simulink model "four_2"  (R2018a)
settings: Solver=VariableStepAuto  StartTime=0.0  StopTime=0.1  RelTol=1e-3
libraries: powerlib x17, powerlib_extras x1
settings Model: Creator=14064  LastModifiedBy=14064

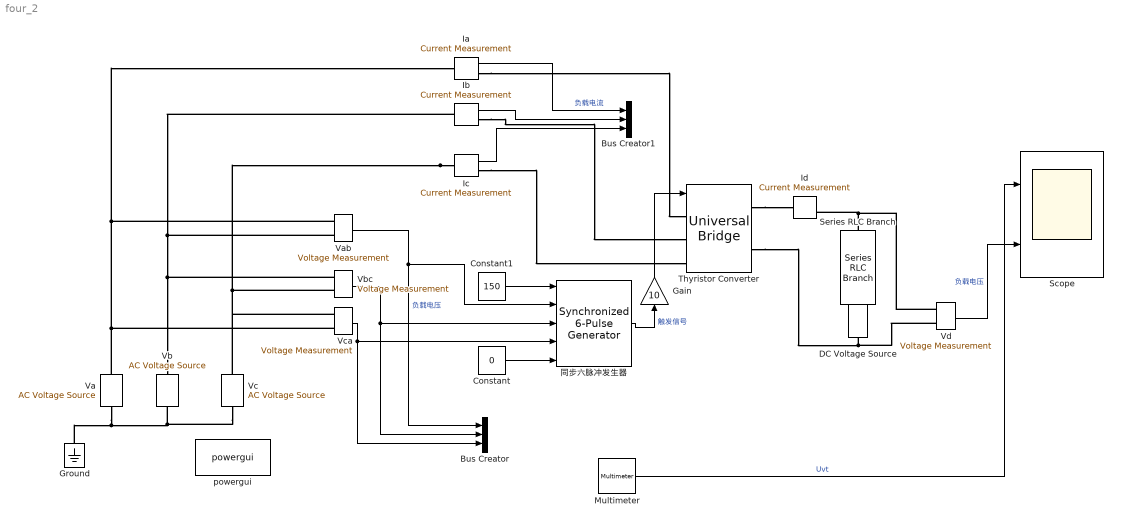
== system four_2 ==
  Bus Creator : BusCreator  Inputs=3
  Bus Creator1 : BusCreator  Inputs=3
  Constant : Constant  Value=0
  Constant1 : Constant  Value=150
  DC Voltage Source : powerlib/Electrical Sources/DC Voltage Source  Amplitude=50  Measurements=None
  Gain : Gain  Gain=10
  Ground : powerlib/Elements/Ground  LConnTagsString=a
  Ia : powerlib/Measurements/Current Measurement  PhasorSimulation=off  OutputType=Complex  PSBequivalent=0
  Ib : powerlib/Measurements/Current Measurement  PhasorSimulation=off  OutputType=Complex  PSBequivalent=0
  Ic : powerlib/Measurements/Current Measurement  PhasorSimulation=off  OutputType=Complex  PSBequivalent=0
  Id : powerlib/Measurements/Current Measurement  PhasorSimulation=off  OutputType=Complex  PSBequivalent=0
  Multimeter : powerlib/Measurements/Multimeter  PhasorSimulation=off  OutputType=Complex  sel=1  L=16  Gain=1  yselected={'Usw1: Thyristor Converter'};  PSBOutputType=1  PSBequivalent=0  AxesSetting=[0,0.1,-100,100]  Display=0  SavedBlockNames=-11
  Scope : Scope  NumInputPorts=2
  Series RLC Branch : powerlib/Elements/Series RLC Branch  LConnTagsString=__new0  RConnTagsString=__new0  BranchType=RL  Resistance=5  Inductance=0.7  SetiL0=off  InitialCurrent=0  Capacitance=inf  Setx0=off  InitialVoltage=0  Measurements=None
  Thyristor Converter : powerlib/Power Electronics/Universal Bridge  Arms=3  SnubberResistance=50  SnubberCapacitance=1e-6  Device=Thyristors  Ron=1e-3  Lon=0  ForwardVoltages="[  0.8  0.8  ]"  ForwardVoltage=0.8  GTOparameters=[ 10e-6 , 20e-6 ]  IGBTparameters=[ 1e-6 , 2e-6 ]  Measurements=All voltages and currents  Measurements_2=None  converterType=Rectifier
  Va : powerlib/Electrical Sources/AC Voltage Source  Amplitude=50  Phase=0  Frequency=50  SampleTime=0  Measurements=None  BusType=swing  Pref=10e3  Qref=0  Qmin=-inf  Qmax=+inf
  Vab : powerlib/Measurements/Voltage Measurement  PhasorSimulation=off  OutputType=Complex  PSBequivalent=0
  Vb : powerlib/Electrical Sources/AC Voltage Source  Amplitude=50  Phase=-120  Frequency=50  SampleTime=0  Measurements=None  BusType=swing  Pref=10e3  Qref=0  Qmin=-inf  Qmax=+inf
  Vbc : powerlib/Measurements/Voltage Measurement  PhasorSimulation=off  OutputType=Complex  PSBequivalent=0
  Vc : powerlib/Electrical Sources/AC Voltage Source  Amplitude=50  Phase=-240  Frequency=50  SampleTime=0  Measurements=None  BusType=swing  Pref=10e3  Qref=0  Qmin=-inf  Qmax=+inf
  Vca : powerlib/Measurements/Voltage Measurement  PhasorSimulation=off  OutputType=Complex  PSBequivalent=0
  Vd : powerlib/Measurements/Voltage Measurement  PhasorSimulation=off  OutputType=Complex  PSBequivalent=0
  powergui : powerlib/powergui  Priority=1  SimulationMode=Continuous  SampleTime=50e-6  frequency=60  Iterations=50  frequencyindice=50  Pbase=100e6  ErrMax=1e-4  UnitsV=kV  UnitsW=MW  buscounter=0  FunctionMessages=off  echomessages=off  EnableUseOfTLC=off  CurrentSourceSwitches=off  DisableSnubberDevices=off  DisableRonSwitches=off  DisableVfSwitches=off  DisplayEquations=off  SolverType=Tustin/Backward Euler (TBE)  Interpol=off  ExternalGateDelay=off  methode=off  Ts=100  x0status=blocks  SPID=on  SwTol=0  HookPort=off  RestoreLinks=warning  ResistiveCurrentMeasurement=off  Frange=[0:2:500]  Ylog=off  Xlog=on  ShowGrid=off  save=off  variable=ZData  structure=0  ZoomFFT=off  StartTime=0.0  cycles=1  DisplayStyle=1  fundamental=60  FreqAxis=off  MaxFrequency=1000  frequencyindicesteady=1  RmsSteady=1  display=off
  同步六脉冲发生器 : powerlib_extras/Control  Blocks/Synchronized 6-Pulse Generator  freq=60  pwidth=10  Double_Pulse=off
  wires:
  Ib/1 -> Bus Creator1/2
  Ia/1 -> Bus Creator1/1  "负载电流"
  Vca/1 -> 同步六脉冲发生器/4, Bus Creator/3
  Vab/1 -> 同步六脉冲发生器/2, Bus Creator/1  "负载电压"
  Vbc/1 -> 同步六脉冲发生器/3, Bus Creator/2
  同步六脉冲发生器/1 -> Gain/1  "触发信号"
  Ic/1 -> Bus Creator1/3
  Constant1/1 -> 同步六脉冲发生器/1
  Constant/1 -> 同步六脉冲发生器/5
  Vd/1 -> Scope/2  "负载电压"
  Gain/1 -> Thyristor Converter/1
  Multimeter/1 -> Scope/1  "Uvt"
  connections:
  Ground/LConn1 -- Va/LConn1 -- Vc/LConn1 -- Vb/LConn1
  Ic/LConn1 -- Vbc/LConn2 -- Vc/RConn1 -- Vca/LConn1
  Vca/LConn2 -- Va/RConn1 -- Vab/LConn1 -- Ia/LConn1
  Ib/LConn1 -- Vab/LConn2 -- Vbc/LConn1 -- Vb/RConn1
  Series RLC Branch/LConn1 -- Vd/LConn1 -- Id/RConn1
  Thyristor Converter/RConn1 -- Id/LConn1
  Ia/RConn1 -- Thyristor Converter/LConn1
  Ic/RConn1 -- Thyristor Converter/LConn3
  Ib/RConn1 -- Thyristor Converter/LConn2
  Thyristor Converter/RConn2 -- Vd/LConn2 -- DC Voltage Source/RConn1
  DC Voltage Source/LConn1 -- Series RLC Branch/RConn1
